simulink model "sim_first_chapter"  (R2019b)
settings: Solver=VariableStepAuto  StartTime=0.0  StopTime=600  RelTol=1e-3
values from neighbouring files (symbols this model uses):
  I = [1 1 1]    [tests_mat.m]
  m = 100    [tests_mat.m]
  n = sqrt(g/R)    [tests_mat.m]
libraries: sharedtransform x2, simulink_extras x1, vrlib x1
settings Model: Creator=asmialek  LastModifiedBy=asmialek

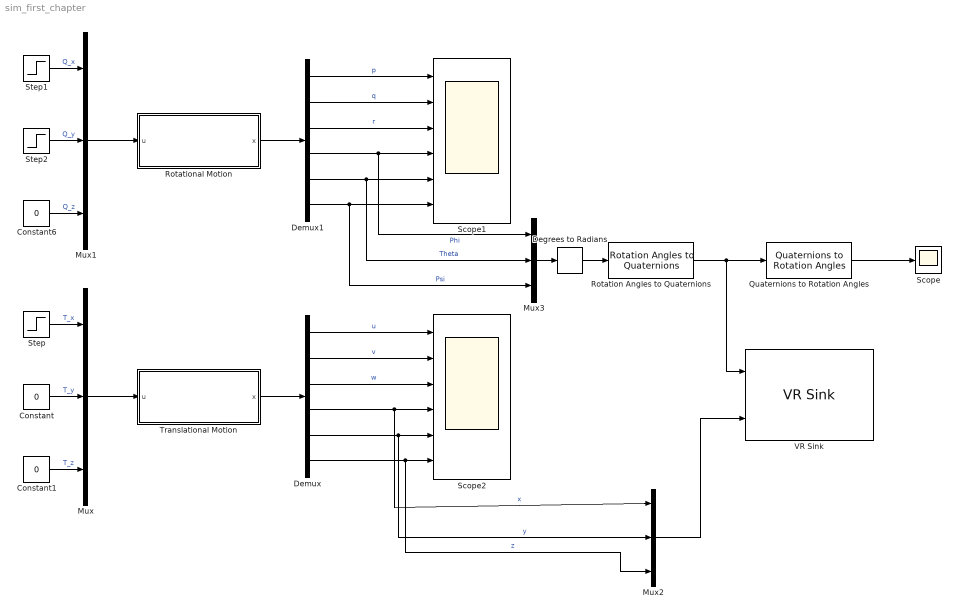
== system sim_first_chapter ==
  Constant : Constant  Value=0
  Constant1 : Constant  Value=0
  Constant6 : Constant  Value=0
  Degrees to Radians : simulink_extras/Transformations/Degrees to Radians
  Demux : Demux  Outputs=6
  Demux1 : Demux  Outputs=6
  Mux{,1..3} (4 alike) : Mux  Inputs=3
  Quaternions to Rotation Angles : sharedtransform/Quaternions to Rotation Angles  rotationOrder=ZYX  aMode=aMode
      settings: SourceProductBaseCode=AE
  Rotation Angles to Quaternions : sharedtransform/Rotation Angles to Quaternions  rotationOrder=XYZ  aMode=aMode
      settings: SourceProductName=Aerospace Blockset  SourceProductBaseCode=AE
  Rotational Motion : Subsystem
  Scope : Scope
  Scope1 : Scope  NumInputPorts=6
  Scope2 : Scope  NumInputPorts=6
  Step : Step  Time=5  After=0.01  SampleTime=0
  Step1 : Step  Time=5  SampleTime=0
  Step2 : Step  Time=15  After=0  SampleTime=0
  Translational Motion : Subsystem
  VR Sink : vrlib/VR Sink  InstantiateOnLoad=on  SampleTime=0.1  ViewEnable=on  RemoteChange=off  RemoteView=off  FieldsWritten=BoxSat.rotation.4.1.1.double#BoxSat.translation.3.1.1.double  WorldFileName=sat_world.wrl  AutoView=off  VideoDimensions=[]  AllowVariableSize=off
      settings: SourceProductName=Simulink
  wires:
  Step/1 -> Mux/1  "T_x"
  Constant/1 -> Mux/2  "T_y"
  Constant1/1 -> Mux/3  "T_z"
  Demux/1 -> Scope2/1  "u"
  Demux/2 -> Scope2/2  "v"
  Demux/3 -> Scope2/3  "w"
  Demux/4 -> Mux2/1, Scope2/4  "x"
  Demux/5 -> Mux2/2, Scope2/5  "y"
  Demux/6 -> Mux2/3, Scope2/6  "z"
  Mux/1 -> Translational Motion/1(u)
  Translational Motion/1(x) -> Demux/1
  Step1/1 -> Mux1/1  "Q_x"
  Demux1/6 -> Mux3/3, Scope1/6  "Psi"
  Demux1/5 -> Mux3/2, Scope1/5  "Theta"
  Demux1/3 -> Scope1/3  "r"
  Demux1/2 -> Scope1/2  "q"
  Demux1/4 -> Mux3/1, Scope1/4  "Phi"
  Demux1/1 -> Scope1/1  "p"
  Step2/1 -> Mux1/2  "Q_y"
  Rotational Motion/1(x) -> Demux1/1
  Constant6/1 -> Mux1/3  "Q_z"
  Mux1/1 -> Rotational Motion/1(u)
  Mux2/1 -> VR Sink/2
  Mux3/1 -> Degrees to Radians/1
  Rotation Angles to Quaternions/1 -> Quaternions to Rotation Angles/1, VR Sink/1
  Degrees to Radians/1 -> Rotation Angles to Quaternions/1
  Quaternions to Rotation Angles/1 -> Scope/1

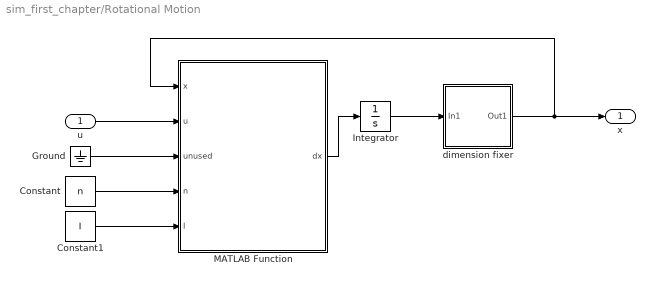
== system sim_first_chapter/Rotational Motion ==
  u : Inport
  Constant : Constant  Value=n
  Constant1 : Constant  Value=I
  Ground : Ground
  Integrator : Integrator
  MATLAB Function : MATLAB Function  TreatAsAtomicUnit=on
  dimension fixer : Subsystem
  x : Outport
  wires:
  Integrator/1 -> dimension fixer/1(In1)
  u/1 -> MATLAB Function/2(u)
  Ground/1 -> MATLAB Function/3(unused)
  MATLAB Function/1(dx) -> Integrator/1
  dimension fixer/1(Out1) -> x/1, MATLAB Function/1(x)
  Constant1/1 -> MATLAB Function/5(I)
  Constant/1 -> MATLAB Function/4(n)

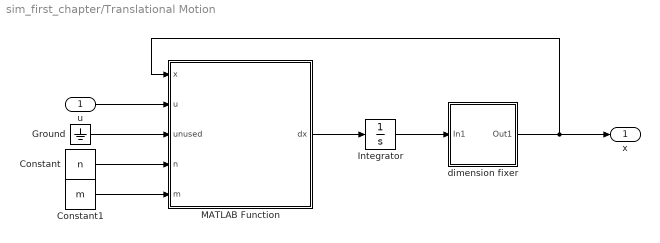
== system sim_first_chapter/Translational Motion ==
  u : Inport
  Constant : Constant  Value=n
  Constant1 : Constant  Value=m
  Ground : Ground
  Integrator : Integrator
  MATLAB Function : MATLAB Function  TreatAsAtomicUnit=on
  dimension fixer : Subsystem
  x : Outport
  wires:
  Integrator/1 -> dimension fixer/1(In1)
  u/1 -> MATLAB Function/2(u)
  Ground/1 -> MATLAB Function/3(unused)
  MATLAB Function/1(dx) -> Integrator/1
  dimension fixer/1(Out1) -> x/1, MATLAB Function/1(x)
  Constant/1 -> MATLAB Function/4(n)
  Constant1/1 -> MATLAB Function/5(m)

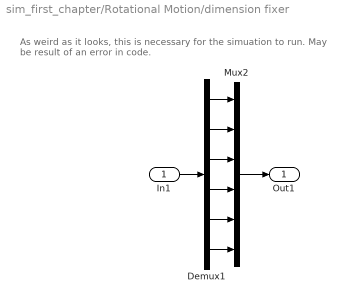
== system sim_first_chapter/Rotational Motion/dimension fixer ==
  note: As weird as it looks, this is necessary for the simuation to run.
      |
      | May be result of an error in code.
  In1 : Inport
  Demux1 : Demux  Outputs=6
  Mux2 : Mux  Inputs=6
  Out1 : Outport
  wires:
  Demux1/1 -> Mux2/1
  Demux1/5 -> Mux2/5
  Demux1/3 -> Mux2/3
  In1/1 -> Demux1/1
  Demux1/6 -> Mux2/6
  Demux1/2 -> Mux2/2
  Demux1/4 -> Mux2/4
  Mux2/1 -> Out1/1

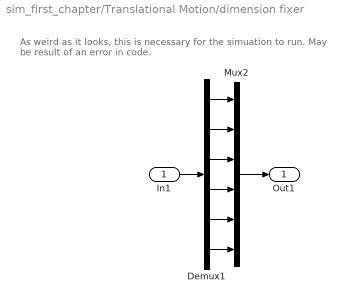
== system sim_first_chapter/Translational Motion/dimension fixer ==
  note: As weird as it looks, this is necessary for the simuation to run.
      |
      | May be result of an error in code.
  In1 : Inport
  Demux1 : Demux  Outputs=6
  Mux2 : Mux  Inputs=6
  Out1 : Outport
  wires:
  Demux1/1 -> Mux2/1
  Demux1/5 -> Mux2/5
  Demux1/3 -> Mux2/3
  In1/1 -> Demux1/1
  Demux1/6 -> Mux2/6
  Demux1/2 -> Mux2/2
  Demux1/4 -> Mux2/4
  Mux2/1 -> Out1/1

== matlab function sim_first_chapter/Rotational Motion/MATLAB Function ==
  data: x input; u input; dx output; unused input; n input; I input
function dx = translational_motion(x, u, ~, n, I)

        p = x(1);
        q = x(2);
        r = x(3);
      phi = x(4);
    theta = x(5);
      psi = x(6);

    G = [ 1  0          -sin(theta)           ;
          0  cos(theta)  cos(theta)*sin(phi)  ;
          0 -sin(theta)  cos(theta)*cos(phi) ];

    F = [ sin(psi)*cos(theta)                               ;
          sin(psi)*sin(theta)*sin(phi) + cos(psi)*cos(phi)  ;
          sin(psi)*sin(theta)*cos(phi) - cos(psi)*sin(phi) ];

%     euler_derivatives = (G^-1)*([p q r]' + F.*n);

    p_dot = (-3*n^2*(I(1) - I(3))*phi + u(1) - n*(I(2) - I(3))*r)/I(1);
    q_dot = (-3*n^2*(I(1) - I(3))*theta + u(2))/I(2);
    r_dot = (u(3) + n*(I(2) - I(1)))/I(3);
    
%     dx = [p_dot; q_dot; r_dot; euler_derivatives];
    
    phi_dot = p + n*psi;
    theta_dot = q + n;
    psi_dot = r - n*phi;
    
    dx = [p_dot; q_dot; r_dot; phi_dot; theta_dot; psi_dot];
end

== matlab function sim_first_chapter/Translational Motion/MATLAB Function ==
  data: x input; u input; dx output; unused input; n input; m input
function dx = translational_motion(x, u, ~, n, m)

    A = [  0   0   n  -n^2 0   0     ;
           0   0   0   0  -n^2 0     ;
          -n   0   0   0   0   2*n^2 ;
           1   0   0   0   0   n     ;
           0   1   0   0   0   0     ;
           0   0   1  -n   0   0    ];

    B = [  1/m 0   0   ;
           0   1/m 0   ;
           0   0   1/m ;
           0   0   0   ;
           0   0   0   ;
           0   0   0  ];   

    dx = A*x + B*u;
end
